simulink model "test_daqbeagle"  (R2014b)
settings: Solver=FixedStepDiscrete  StartTime=0.0  StopTime=Inf  FixedStep=0.01  RelTol=1e-3
StartFcn:
  | run runtarget
libraries: simulink x1
settings Model: SimulationMode=external  ExtModeTrigDuration=100000  Creator=parallels  LastModifiedBy=parallels
settings OptimizationCC: OptimizeModelRefInitCode=on  LifeSpan=Inf
settings RTWCC: SystemTargetFile=ert_linux.tlc  MakeCommand="make_rtw CC=arm-linux-gnueabihf-gcc CPP=arm-linux-gnueabihf-g++ OPTS=\"-DWITH_HW -DUSE_STARTUP_FILE\" OPTIMIZATION_FLAGS=-O3 ADDITIONAL_LDFLAGS=\"-static -static-libgcc\""  TemplateMakefile=ert_linux.tmf  Description=Linux Embedded Coder  ProcessScript=ert_linux_make_rtw_hook  TargetLang=C++
settings CodeAppCC: IgnoreCustomStorageClasses=off
settings STFCustomTargetCC: ModelReferenceCompliant=off  CombineOutputUpdateFcns=on  ERTCustomFileBanners=on  SupportAbsoluteTime=off  SupportNonFinite=off  SupportComplex=off  SupportContinuousTime=off  SupportNonInlinedSFcns=off  MATLABClassNameForMDSCustomization=Simulink.SoftwareTarget.ERTCustomization  GRTInterface=off  SystemTargetFile=ert_linux.tlc
settings ERTTargetCC: ModelReferenceCompliant=off  ParMdlRefBuildCompliant=off  CompOptLevelCompliant=off  ConcurrentExecutionCompliant=off  ERTFirstTimeCompliant=off  SupportAbsoluteTime=off  SupportNonFinite=off  SupportComplex=off  ModelStepFunctionPrototypeControlCompliant=off  CPPClassGenCompliant=off  ExtMode=on  ExtModeMexArgs='192.168.7.2' 1 17725  InlinedParameterPlacement=NonHierarchical  ERTCustomFileTemplate=ert_linux_file_process.tlc

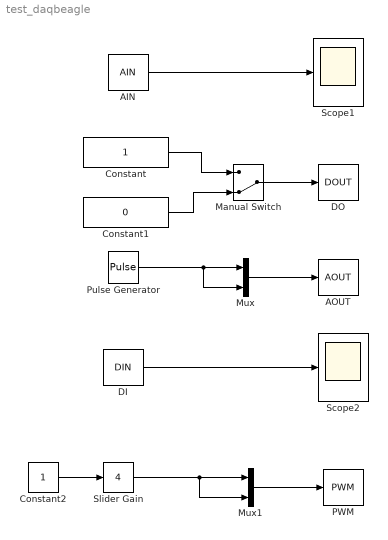
== system test_daqbeagle ==
  AIN : S-Function  FunctionName=AIN  Parameters=sampleTime  EnableBusSupport=off  mask{sampleTime=0.01}
      mask prompts: sampleTime "Enter sample time"
      mask DialogControl Control2 Prompt: This block uses a memory map to access the 7 ADC channels of the beaglebone black. The output is a vector of size 7 with a amplitude range of 0..4095. Fullscale means 1.8V and 0 GND.
      mask Display:
      | pos = get_param(gcb, 'Position');
      | width = pos(3) - pos(1);
      | height = pos(4) - pos(2);
      | x = [0, width];
      | y = [0, height];
      | plot(x,y)
      | text(0.25*width, 0.75*height,'A');
      | text(0.75*width, 0.25*height,'D');
  AOUT : S-Function  FunctionName=AOUT  Parameters=sampleTime  EnableBusSupport=off  mask{sampleTime=0.01}
      mask prompts: sampleTime "Enter sample time"
      mask DialogControl Control2 Prompt: This block uses a memory map to access the 2 DAC channels of the beaglebone black. The input is a vector of size 2 with a amplitude range of 0..5V.
      mask Display:
      | pos = get_param(gcb, 'Position');
      | width = pos(3) - pos(1);
      | height = pos(4) - pos(2);
      | x = [0, width];
      | y = [0, height];
      | plot(x,y)
      | text(0.25*width, 0.75*height,'D');
      | text(0.75*width, 0.25*height,'A');
  Constant : Constant  OutDataTypeStr=uint8
  Constant1 : Constant  Value=0  OutDataTypeStr=uint8
  Constant2 : Constant
  DI : S-Function  FunctionName=DIN  Parameters=uint8(pinEnable), sampleTime  EnableBusSupport=off  mask{pinEnable=[6 7 8], sampleTime=0.01}
      mask prompts: pinEnable "Please enter channel vector."; sampleTime "Enter sample time"
      mask init:
      | if (~issorted(pinEnable)) 
      |     error('Vector has to be in ascending order');
      |     pinEnable = sort(pinEnable);
      | end
      | 
      | if (unique(pinEnable) ~= pinEnable)
      |     error('There are duplicates inside the vector');
      |     pinEnable = unique(pinEnable);
      | end
      | 
      | if (length(pinEnable) > 8)
      |     error('Vector has more than 8 elements');
      |     pinEnable = pinEnable(1:8);
      | end
      | 
      | if ((max(pinEnable) > 8) || (min(pinEnable) < 1))
      |     error('All channels have to be in the range 1..8');
      |     pinEnable = pinEnable(find((pinEnable >= 8) && (pinEnable >= 1)));
      | end
      mask DialogControl Control2 Prompt: This block uses a memory map to access 8 GPIO as input. The block outputs a vector of 8 uint8 values. The value for each channels will be  0 for a logic LOW or 1 for a logic HIGH. If a startup script for exporting all pins is used the compile flag USE_STARTUP_FILE has to be added to the make command inside configuration. Please enter the pins you want to enable. The vector should ascending order and without doublicats. The maximum number should be 8 and the minimum 1.
      mask Display: disp('DI')
  DO : S-Function  FunctionName=DOUT  Parameters=uint8(pinEnable), sampleTime  EnableBusSupport=off  mask{pinEnable=[8], sampleTime=0.01}
      mask prompts: pinEnable "Please enter channel vector."; sampleTime "Enter sample time"
      mask init: same as test_daqbeagle/DI
      mask DialogControl Control2 Prompt: This block uses a memory map to access 8 GPIO as output. The block accepts an input vector of 8 uint8 values. The value has to be 0 for a logic LOW or 1 for a logic HIGH. If a startup script for exporting all pins is used the compile flag USE_STARTUP_FILE has to be added to the make command inside configuration. Please enter the pins you want to enable. The vector should ascending order and without doublets. The maximum number should be 8 and the minimum 1.
      mask Display: disp('DO')
  Manual Switch : ManualSwitch  CurrentSetting=0
  Mux : Mux  Inputs=2
  Mux1 : Mux  Inputs=2
  PWM : S-Function  FunctionName=PWM  Parameters=frequency, sampleTime  EnableBusSupport=off  mask{frequency=1E5, sampleTime=0.01}
      mask prompts: frequency "Enter the frequency of the PWM module"; sampleTime "Enter sample time"
      mask DialogControl Control2 Prompt: This block uses a memory map to access the 2 PWM channels of the beaglebone black. The input is a vector of size 2 with a amplitude range of 0..100%.
      mask Display: disp('PWM')
  Pulse Generator : DiscretePulseGenerator  Amplitude=5  Period=200  PulseWidth=100  SampleTime=0.01
  Scope1 : Scope
      settings: TimeRange=10  YMin=0  YMax=600
  Scope2 : Scope
      settings: TimeRange=10  YMin=-0.1  YMax=1.1
  Slider Gain : simulink/Math Operations/Slider Gain  low=0  gain=4  high=100
  wires:
  AIN/1 -> Scope1/1
  Constant/1 -> Manual Switch/1
  Constant1/1 -> Manual Switch/2
  Manual Switch/1 -> DO/1
  DI/1 -> Scope2/1
  Pulse Generator/1 -> Mux/2, Mux/1
  Mux/1 -> AOUT/1
  Constant2/1 -> Slider Gain/1
  Mux1/1 -> PWM/1
  Slider Gain/1 -> Mux1/1, Mux1/2
